simulink model "longitudinal_model"  (R2025a)
settings: Solver=ode45  StartTime=0.0  StopTime=2500  RelTol=1e-3
values from neighbouring files (symbols this model uses):
  m = 1500    [drivetrain.m]    (also in project_parameters.m = 1400)
libraries: autolibshared x1
settings Model: Creator=DELL  LastModifiedBy=DELL

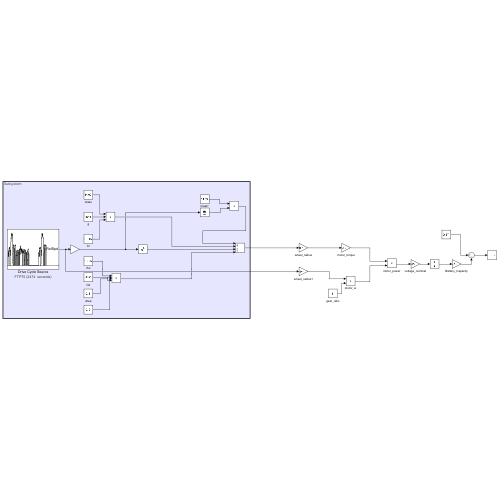
[thumbnail: Simulink's stored preview of the top-level diagram]
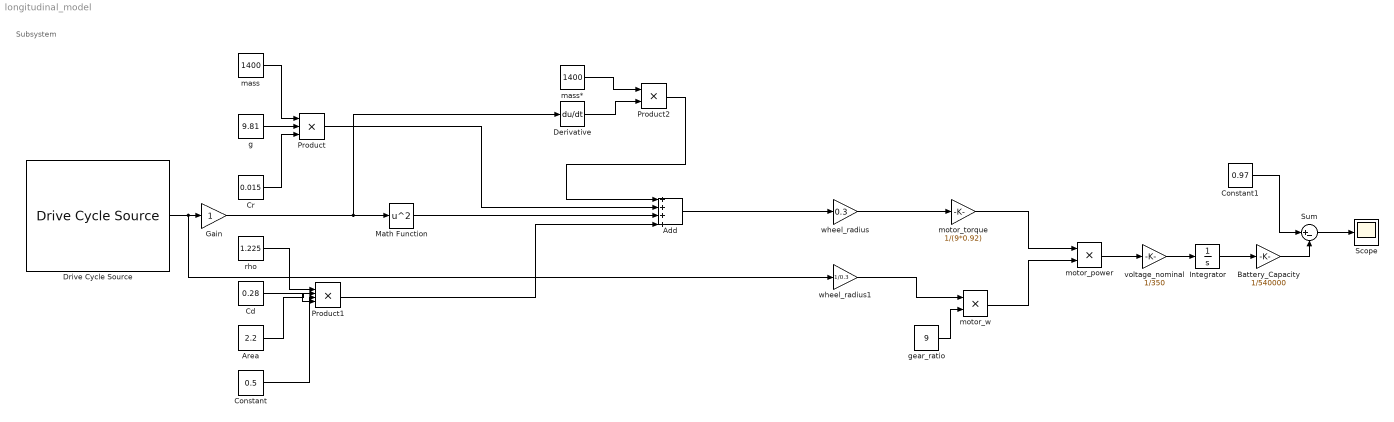
== system longitudinal_model ==
  note: Subsystem
  Add : Sum  Inputs=++++
  Area : Constant  Value=2.2
  Battery_Capacity : Gain  Gain=1/540000
  Cd : Constant  Value=0.28
  Constant : Constant  Value=0.5
  Constant1 : Constant  Value=0.97
  Cr : Constant  Value=0.015
  Derivative : Derivative
  Drive Cycle Source : autolibshared/Drive Cycle Source  cycleVar=FTP75  fileVar=cycleFTP75.mat  tfinal="2474  seconds"  cycleRepeat=off  outAccPort=off  outGearPort=off  gearList=No gear data  t_wot1=5  xdot_woto=0  xdot_wot1=30  t_wot2=20  xdot_wot2=0  t_wotend=30  srcUnit=m/s  outUnit=m/s  srcAccUnit=m/s/s  outAccUnit=m/s^2  dt=0  aMode=1  faultOption=off  velBnd=2  velBndUnit=mph  inUnit=m/s  timeBnd=1  failOption=off  stopSim=off  maxFaultCnt=10  maxFaultTime=2  maxTotFaultTime=15  traceOption=off  dtTrace=1  traceWindow=10  lastDCname=FTP75  lastOutUnit=mph  lastDT=0  lastTB=1  lastSB=2  forceCalcBound=off
  Gain : Gain
  Integrator : Integrator
  Math Function : Math  Operator=square
  Product : Product  Inputs=3
  Product1 : Product  Inputs=4
  Product2 : Product
  Scope : Scope
      settings: ActiveDisplayYMinimum=0.9157345544716885  ActiveDisplayYMaximum=0.9760294939475902
  Sum : Sum  Inputs=|+-
  g : Constant  Value=9.81
  gear_ratio : Constant  Value=9
  mass : Constant  Value=1400
  mass* : Constant  Value=1400
  motor_power : Product
  motor_torque : Gain  Gain=1/(9*0.92)
  motor_w : Product
  rho : Constant  Value=1.225
  voltage_nominal : Gain  Gain=1/350
  wheel_radius : Gain  Gain=0.3
  wheel_radius1 : Gain  Gain=1/0.3
  wires:
  Add/1 -> wheel_radius/1
  Area/1 -> Product1/2
  Cr/1 -> Product/3
  Cd/1 -> Product1/4
  Product2/1 -> Add/1
  Math Function/1 -> Add/3
  mass/1 -> Product/1
  Product/1 -> Add/2
  Drive Cycle Source/1 -> wheel_radius1/1, Gain/1
  Product1/1 -> Add/4
  Constant/1 -> Product1/3
  g/1 -> Product/2
  rho/1 -> Product1/1
  Derivative/1 -> Product2/2
  Gain/1 -> Derivative/1, Math Function/1
  mass*/1 -> Product2/1
  wheel_radius/1 -> motor_torque/1
  wheel_radius1/1 -> motor_w/1
  gear_ratio/1 -> motor_w/2
  motor_torque/1 -> motor_power/1
  motor_w/1 -> motor_power/2
  Integrator/1 -> Battery_Capacity/1
  Constant1/1 -> Sum/1
  Battery_Capacity/1 -> Sum/2
  motor_power/1 -> voltage_nominal/1
  voltage_nominal/1 -> Integrator/1
  Sum/1 -> Scope/1
